simulink library "wt_blockset_beta"  (Simulink 5.0)
values from neighbouring files (symbols this model uses):
  a = -Le\Re    [matrix_coeff_trafo3limb_abc.m]
  a11 = K2*Rs/Ls    [matrix_coeff_scim_abc.m]    (also in matrix_coeff_spsm_dq.m = -Rs*Ksgm_frd/Ksgm_d; matrix_coeff_trafo_abc.m = K2*Rhv/Lhv; matrix_coeff_wrim_abc.m)
  a12 = K3*Rs/Ls    [matrix_coeff_scim_abc.m]    (also in matrix_coeff_spsm_dq.m = Lssq*Ksgm_frd/Ksgm_d; matrix_coeff_trafo_abc.m = K3*Rhv/Lhv; matrix_coeff_wrim_abc.m)
  a13 = 3*Msr*sqrt(3)*K4/4    [matrix_coeff_scim_abc.m]    (also in matrix_coeff_spsm_dq.m = Rf*Lsgm_rd*Lmd/Ksgm_d; matrix_coeff_trafo_abc.m = K4*Rhv; matrix_coeff_wrim_abc.m)
  a14 = K4*Rr    [matrix_coeff_scim_abc.m]    (also in matrix_coeff_spsm_dq.m = Rrd*Lsgm_f*Lmd/Ksgm_d; matrix_coeff_trafo_abc.m = K2/Lhv; matrix_coeff_wrim_abc.m)
  a15 = Msr*(K2-K3)/Ls    [matrix_coeff_scim_abc.m]    (also in matrix_coeff_spsm_dq.m = Lmq*Ksgm_frd/Ksgm_d; matrix_coeff_trafo_abc.m = K3/Lhv; matrix_coeff_wrim_abc.m)
  a16 = K2/Ls    [matrix_coeff_scim_abc.m]    (also in matrix_coeff_spsm_dq.m = Ksgm_frd/Ksgm_d; matrix_coeff_trafo_abc.m = K4; matrix_coeff_wrim_abc.m)
  a17 = K3/Ls    [matrix_coeff_scim_abc.m]    (also in matrix_coeff_spsm_dq.m = -Lsgm_rd*Lmd/Ksgm_d; matrix_coeff_wrim_abc.m)
  a21 = -Lssd*Lsrq/Ksgm_q    [matrix_coeff_spsm_dq.m]
  a22 = -Rs*Lsrq/Ksgm_q    [matrix_coeff_spsm_dq.m]
  a23 = -Lsrq*Lmd/Ksgm_q    [matrix_coeff_spsm_dq.m]
  a24 = -Lsrq*Lmd/Ksgm_q    [matrix_coeff_spsm_dq.m]
  a25 = Rrq*Lmq/Ksgm_q    [matrix_coeff_spsm_dq.m]
  a26 = Lsrq/Ksgm_q    [matrix_coeff_spsm_dq.m]
  a31 = K4*Rs    [matrix_coeff_scim_abc.m]    (also in matrix_coeff_spsm_dq.m = +Rs*Lsgm_rd*Lmd/Ksgm_d; matrix_coeff_trafo_abc.m = K4*Rlv; matrix_coeff_wrim_abc.m)
  a32 = Msr*(K2-K3)/Lr    [matrix_coeff_scim_abc.m]    (also in matrix_coeff_spsm_dq.m = -Lssq*Lsgm_rd*Lmd/Ksgm_d; matrix_coeff_trafo_abc.m = K2*Rlv/Llv; matrix_coeff_wrim_abc.m)
  a33 = K2*Rr/Lr    [matrix_coeff_scim_abc.m]    (also in matrix_coeff_spsm_dq.m = -Rf*Ksgm_srd/Ksgm_d; matrix_coeff_trafo_abc.m = K3*Rlv/Llv; matrix_coeff_wrim_abc.m)
  a34 = K3*Rr/Lr    [matrix_coeff_scim_abc.m]    (also in matrix_coeff_spsm_dq.m = Rrd*Lsgm_s*Lmd/Ksgm_d; matrix_coeff_trafo_abc.m = K4; matrix_coeff_wrim_abc.m)
  a35 = 3*Msr*sqrt(3)*K4/4    [matrix_coeff_scim_abc.m]    (also in matrix_coeff_spsm_dq.m = -Lsgm_rd*Lmd*Lmq/Ksgm_d; matrix_coeff_trafo_abc.m = K2/Llv; matrix_coeff_wrim_abc.m)
  a36 = K4    [matrix_coeff_scim_abc.m]    (also in matrix_coeff_spsm_dq.m = -Lsgm_rd*Lmd/Ksgm_d; matrix_coeff_trafo_abc.m = K3/Llv; matrix_coeff_wrim_abc.m)
  a37 = Ksgm_srd/Ksgm_d    [matrix_coeff_spsm_dq.m]    (also in matrix_coeff_wrim_abc.m = K2/Lr)
  a41 = Rs*Lsgm_f*Lmd/Ksgm_d    [matrix_coeff_spsm_dq.m]
  a42 = -Lsgm_f*Lssq*Lmd/Ksgm_d    [matrix_coeff_spsm_dq.m]
  a43 = Rf*Lsgm_s*Lmd/Ksgm_d    [matrix_coeff_spsm_dq.m]
  a44 = -Rrd*Ksgm_sf/Ksgm_d    [matrix_coeff_spsm_dq.m]
  a45 = -Lsgm_f*Lmd*Lmq/Ksgm_d    [matrix_coeff_spsm_dq.m]
  a46 = -Lsgm_f*Lmd/Ksgm_d    [matrix_coeff_spsm_dq.m]
  a47 = -Lsgm_s*Lmd/Ksgm_d    [matrix_coeff_spsm_dq.m]
  a51 = Lssd*Lmq/Ksgm_q    [matrix_coeff_spsm_dq.m]
  a52 = Rs*Lmq/Ksgm_q    [matrix_coeff_spsm_dq.m]
  a53 = Lmd*Lmq/Ksgm_q    [matrix_coeff_spsm_dq.m]
  a54 = Lmd*Lmq/Ksgm_q    [matrix_coeff_spsm_dq.m]
  a55 = -Rrq*Lssq/Ksgm_q    [matrix_coeff_spsm_dq.m]
  a56 = -Lmq/Ksgm_q    [matrix_coeff_spsm_dq.m]
  alpha_T = Ubase_hv/Ubase_lv    [matrix_coeff_trafo3limb_abc.m]
  b = inv(Le)    [matrix_coeff_trafo3limb_abc.m]
  Ctorque = cq(2:5:102,2:5:182)    [cq_table.m]
  Lmd = mag_ind(1)    [matrix_coeff_spsm_dq.m]
  Lmq = mag_ind(2)    [matrix_coeff_spsm_dq.m]
  Lss = Lsgms+Lm    [init_dbe_dq_scim.m]
  omg_base = 2*pi*rated_fp(1)    [init_dbe_dq_scim.m]    (also in init_dbe_rms_scim.m)
  p = rated_fp(2)    [init_dbe_dq_scim.m]    (also in init_dbe_rms_scim.m)
  Rs = stator(1)    [init_dbe_dq_scim.m]    (also in init_dbe_rms_scim.m; matrix_coeff_scim_abc.m; matrix_coeff_spsm_dq.m = stator_winding(1); matrix_coeff_wrim_abc.m)
  Xs = omg_base*Lss    [init_dbe_dq_scim.m]    (also in init_dbe_rms_scim.m = Xsgm_s+Xm)
undefined symbols (not defined in the file or in its folder): get, j, Kmode, ModeOp, Type, u0
libraries: simulink_extras x12, simulink x4, dspinverses x1, dspmtrx3 x1, dspsigattribs x1, dspspect3 x1
(part 3 of 4)

== system wt_blockset_beta/Mechanical Components/Wind Model SB-2/3rd_Harmonic_Filter2 ==
  avg_wind : Inport
  in_1 : Inport  Port=2
  3rd harmonic Filter : Subsystem
  Unit Delay : UnitDelay  SampleTime=T_sample
  out_1 : Outport
  wires:
  3rd harmonic Filter/1(Out) -> out_1/1
  avg_wind/1 -> 3rd harmonic Filter/1(avg_wind)
  in_1/1 -> Unit Delay/1
  Unit Delay/1 -> 3rd harmonic Filter/2(In)

== system wt_blockset_beta/Mechanical Components/Wind Model SB-2/Kaimal_Filter_1 ==
  in_1 : Inport
  avg_wind : Inport  Port=2
  Fcn : Fcn  Expr=turb_int*sqrt(L*u(1))/100/sqrt(2)
  Kaimal Filter : Subsystem
  Product : Product  SaturateOnIntegerOverflow=on
  Unit Delay : UnitDelay  SampleTime=T_sample
  out_1 : Outport
  wires:
  Unit Delay/1 -> Kaimal Filter/2(In)
  in_1/1 -> Unit Delay/1
  avg_wind/1 -> Kaimal Filter/1(avg_wind), Fcn/1
  Fcn/1 -> Product/1
  Kaimal Filter/1(Out) -> Product/2
  Product/1 -> out_1/1

== system wt_blockset_beta/Mechanical Components/Wind Model SB-2/Kaimal_Filter_2 ==
  avg_wind : Inport
  in_1 : Inport  Port=2
  Fcn : Fcn  Expr=turb_int*sqrt(L*u(1))/100/sqrt(2)
  Kaimal Filter : Subsystem
  Product : Product  SaturateOnIntegerOverflow=on
  Unit Delay : UnitDelay  SampleTime=T_sample
  out_1 : Outport
  wires:
  Product/1 -> out_1/1
  Kaimal Filter/1(Out) -> Product/2
  Fcn/1 -> Product/1
  avg_wind/1 -> Fcn/1, Kaimal Filter/1(avg_wind)
  in_1/1 -> Unit Delay/1
  Unit Delay/1 -> Kaimal Filter/2(In)

== system wt_blockset_beta/Mechanical Components/Wind Model SB-2/Kaimal_Filter_3 ==
  avg_wind : Inport
  in_1 : Inport  Port=2
  Fcn : Fcn  Expr=turb_int*sqrt(L*u(1))/100/sqrt(2)
  Kaimal Filter : Subsystem
  Product : Product  SaturateOnIntegerOverflow=on
  Unit Delay : UnitDelay  SampleTime=T_sample
  out_1 : Outport
  wires:
  Unit Delay/1 -> Kaimal Filter/2(In)
  in_1/1 -> Unit Delay/1
  avg_wind/1 -> Kaimal Filter/1(avg_wind), Fcn/1
  Fcn/1 -> Product/1
  Kaimal Filter/1(Out) -> Product/2
  Product/1 -> out_1/1

== system wt_blockset_beta/Mechanical Components/Wind Model SB-2/White Noise_1 ==
  Gain : Gain  Gain=[sqrt(Cov)]/[sqrt(Ts)]  SaturateOnIntegerOverflow=on
  White Noise : RandomNumber  Seed=seed  SampleTime=Ts
  Zero-Order Hold : ZeroOrderHold  SampleTime=Ts
  Out_1 : Outport
  wires:
  Zero-Order Hold/1 -> Gain/1
  Gain/1 -> Out_1/1
  White Noise/1 -> Zero-Order Hold/1

== system wt_blockset_beta/Mechanical Components/Wind Model SB-2/White Noise_2 ==
  Gain : Gain  Gain=[sqrt(Cov)]/[sqrt(Ts)]  SaturateOnIntegerOverflow=on
  White Noise : RandomNumber  Seed=seed  SampleTime=Ts
  Zero-Order Hold : ZeroOrderHold  SampleTime=Ts
  Out_1 : Outport
  wires:
  Zero-Order Hold/1 -> Gain/1
  Gain/1 -> Out_1/1
  White Noise/1 -> Zero-Order Hold/1

== system wt_blockset_beta/Mechanical Components/Wind Model SB-2/White Noise_3 ==
  Gain : Gain  Gain=[sqrt(Cov)]/[sqrt(Ts)]  SaturateOnIntegerOverflow=on
  White Noise : RandomNumber  Seed=seed  SampleTime=Ts
  Zero-Order Hold : ZeroOrderHold  SampleTime=Ts
  Out_1 : Outport
  wires:
  Zero-Order Hold/1 -> Gain/1
  Gain/1 -> Out_1/1
  White Noise/1 -> Zero-Order Hold/1

== system wt_blockset_beta/Mechanical Components/Wind Model SB-2/ZERO_Harmonic_Filter ==
  in_1 : Inport
  avg_wind : Inport  Port=2
  Unit Delay : UnitDelay  SampleTime=T_sample
  ZERO harmonic Filter : Subsystem
  out_1 : Outport
  wires:
  ZERO harmonic Filter/1(Out) -> out_1/1
  avg_wind/1 -> ZERO harmonic Filter/1(avg_wind)
  in_1/1 -> Unit Delay/1
  Unit Delay/1 -> ZERO harmonic Filter/2(In)

== system wt_blockset_beta/Power Converters/3-phase Diode Bridge Rectifier/Diode  State Calculator ==
  note: K = [d1 - d4
      |        d3 - d6
      |         d5 - d2]
  RST : Inport
  Branch A+ : Subsystem
  Branch A- : Subsystem
  Branch B+ : Subsystem
  Branch B- : Subsystem
  Branch C+ : Subsystem
  Branch C- : Subsystem
  Mux : Mux  Inputs=3
  Sum : Sum  Inputs=+-  SaturateOnIntegerOverflow=on  InputSameDT=on
  Sum1 : Sum  Inputs=+-  SaturateOnIntegerOverflow=on  InputSameDT=on
  Sum2 : Sum  Inputs=+-  SaturateOnIntegerOverflow=on  InputSameDT=on
  K : Outport  InitialOutput=0
  wires:
  RST/1 -> Branch A+/1(RST), Branch B+/1(RST), Branch B-/1(RST), Branch C+/1(RST), Branch C-/1(RST), Branch A-/1(RST)
  Branch A+/1(A) -> Sum/1
  Branch A-/1(A) -> Sum/2
  Branch B+/1(B) -> Sum1/1
  Branch B-/1(B) -> Sum1/2
  Branch C+/1(C) -> Sum2/1
  Branch C-/1(C) -> Sum2/2
  Sum/1 -> Mux/1
  Sum1/1 -> Mux/2
  Sum2/1 -> Mux/3
  Mux/1 -> K/1

== system wt_blockset_beta/Power Converters/Average SVM Strategy/1st quadrant ==
  note: 1st quadrant
  vd : Inport
  vq : Inport  Port=2
  Action Port : ActionPort  InitializeStates=reset
  Gain : Gain  Gain=sqrt(3)  SaturateOnIntegerOverflow=on
  If : If  NumInputs=2  IfExpression=u2 < u1
  Sector 0 : Subsystem  TreatAsAtomicUnit=on
  Sector 1 : Subsystem  TreatAsAtomicUnit=on
  Sum : Sum  Inputs=+|+  SaturateOnIntegerOverflow=on
  duty_ABC : Outport  OutputWhenDisabled=reset  InitialOutput=[0 0 0]
  wires:
  vd/1 -> Gain/1, [vd]
  vq/1 -> If/2, [vq]
  Gain/1 -> If/1
  If/1 -> Sector 0/Action
  [vd] -> Sector 0/1(vd)
  [vq] -> Sector 0/2(vq)
  If/2 -> Sector 1/Action
  [vd] -> Sector 1/1(vd)
  [vq] -> Sector 1/2(vq)
  Sector 1/1(duty_ABC) -> Sum/2
  Sector 0/1(duty_ABC) -> Sum/1
  Sum/1 -> duty_ABC/1

== system wt_blockset_beta/Power Converters/Average SVM Strategy/2nd quadrant ==
  note: 2nd quadrant
  vd : Inport
  vq : Inport  Port=2
  Action Port : ActionPort  InitializeStates=reset
  Abs : Abs  SaturateOnIntegerOverflow=on
  Gain : Gain  Gain=sqrt(3)  SaturateOnIntegerOverflow=on
  If : If  NumInputs=2  IfExpression=u2 < u1
  Sector 1 : Subsystem  TreatAsAtomicUnit=on
  Sector 2 : Subsystem  TreatAsAtomicUnit=on
  Sum : Sum  Inputs=+|+  SaturateOnIntegerOverflow=on
  duty_ABC : Outport  OutputWhenDisabled=reset  InitialOutput=[0 0 0]
  wires:
  Sum/1 -> duty_ABC/1
  Sector 2/1(duty_ABC) -> Sum/1
  Sector 1/1(duty_ABC) -> Sum/2
  [vq] -> Sector 1/2(vq)
  [vd] -> Sector 1/1(vd)
  If/2 -> Sector 1/Action
  [vq] -> Sector 2/2(vq)
  [vd] -> Sector 2/1(vd)
  If/1 -> Sector 2/Action
  vq/1 -> [vq], If/2
  vd/1 -> [vd], Abs/1
  Gain/1 -> If/1
  Abs/1 -> Gain/1

== system wt_blockset_beta/Power Converters/Average SVM Strategy/3rd quadrant ==
  note: 3rd quadrant
  vd : Inport
  vq : Inport  Port=2
  Action Port : ActionPort  InitializeStates=reset
  Abs : Abs  SaturateOnIntegerOverflow=on
  Abs1 : Abs  SaturateOnIntegerOverflow=on
  Gain : Gain  Gain=sqrt(3)  SaturateOnIntegerOverflow=on
  If : If  NumInputs=2  IfExpression=u2 <= u1
  Sector 3 : Subsystem  TreatAsAtomicUnit=on
  Sector 4 : Subsystem  TreatAsAtomicUnit=on
  Sum : Sum  Inputs=+|+  SaturateOnIntegerOverflow=on
  duty_ABC : Outport  OutputWhenDisabled=reset  InitialOutput=[0 0 0]
  wires:
  Sum/1 -> duty_ABC/1
  Sector 3/1(duty_ABC) -> Sum/1
  Sector 4/1(duty_ABC) -> Sum/2
  [vq] -> Sector 4/2(vq)
  [vd] -> Sector 4/1(vd)
  If/2 -> Sector 4/Action
  [vq] -> Sector 3/2(vq)
  [vd] -> Sector 3/1(vd)
  If/1 -> Sector 3/Action
  vq/1 -> [vq], Abs1/1
  vd/1 -> [vd], Abs/1
  Gain/1 -> If/1
  Abs/1 -> Gain/1
  Abs1/1 -> If/2

== system wt_blockset_beta/Power Converters/Average SVM Strategy/4th quadrant ==
  note: 4th quadrant
  vd : Inport
  vq : Inport  Port=2
  Action Port : ActionPort  InitializeStates=reset
  Abs1 : Abs  SaturateOnIntegerOverflow=on
  Gain : Gain  Gain=sqrt(3)  SaturateOnIntegerOverflow=on
  If : If  NumInputs=2  IfExpression=u2 <= u1
  Sector 4 : Subsystem  TreatAsAtomicUnit=on
  Sector 5 : Subsystem  TreatAsAtomicUnit=on
  Sum : Sum  Inputs=+|+  SaturateOnIntegerOverflow=on
  duty_ABC : Outport  OutputWhenDisabled=reset  InitialOutput=[0 0 0]
  wires:
  Abs1/1 -> If/2
  vd/1 -> [vd], Gain/1
  vq/1 -> Abs1/1, [vq]
  If/1 -> Sector 5/Action
  [vd] -> Sector 5/1(vd)
  [vq] -> Sector 5/2(vq)
  If/2 -> Sector 4/Action
  [vd] -> Sector 4/1(vd)
  [vq] -> Sector 4/2(vq)
  Sector 4/1(duty_ABC) -> Sum/2
  Sector 5/1(duty_ABC) -> Sum/1
  Sum/1 -> duty_ABC/1
  Gain/1 -> If/1

== system wt_blockset_beta/Power Converters/Average SVM Strategy/Avoid saturation  ==
  Mux : Mux  Inputs=7
  Sign_vdref : Signum
  Sign_vqref : Signum
  vd : Fcn  Expr=(abs(u[1])>u[6])*((3*u(2)*u[6])/(2*u[5]))+(abs(u[1])<=u[6])*(3*u[1]/2/u[5])
  vq : Fcn  Expr=(abs(u[3])>u[7])*((3*u(4)*u[7])/(2*u[5]))+(abs(u[3])<=u[7])*(3*u[3]/2/u[5])
  tag scope: vd=global, vq=global
  wires:
  [vdref] -> Mux/1, Sign_vdref/1
  Mux/1 -> vd/1, vq/1
  vd/1 -> [vd]
  vq/1 -> [vq]
  Sign_vdref/1 -> Mux/2
  [vqref] -> Mux/3, Sign_vqref/1
  Sign_vqref/1 -> Mux/4
  [vdc] -> Mux/5
  [dlim] -> Mux/6
  [qlim] -> Mux/7

== system wt_blockset_beta/Power Converters/Average SVM Strategy/Weight ==
  Abs : Abs  SaturateOnIntegerOverflow=on
  "Abs " : Abs  SaturateOnIntegerOverflow=on
  Mux : Mux  Inputs=3
  Product : Product  SaturateOnIntegerOverflow=on
  Product1 : Product  SaturateOnIntegerOverflow=on
  weight : Fcn  Expr=u(2)/(sqrt(3)*sqrt(u(1)^2+u(3)^2))
  tag scope: dlim=global, qlim=global
  wires:
  [vdref] -> Mux/1, Product/1
  Mux/1 -> weight/1
  [vdc] -> Mux/2
  [vqref] -> Mux/3, Product1/2
  weight/1 -> Product/2, Product1/1
  Product/1 -> Abs/1
  Product1/1 -> "Abs "/1
  Abs/1 -> [dlim]
  "Abs "/1 -> [qlim]

== system wt_blockset_beta/Power Converters/Average SVM Strategy/capcom duty cycle ==
  duty_ABC : Inport
  Constant : Constant  Value=0.5
  Sum : Sum  Inputs=|+-  SaturateOnIntegerOverflow=on
  pwm_abc : Outport
  wires:
  Constant/1 -> Sum/2
  Sum/1 -> pwm_abc/1
  duty_ABC/1 -> Sum/1

== system wt_blockset_beta/Power Converters/Switching PWM Strategy/capcom ==
  duty_abc : Inport
  Reshape : simulink/Math Operations/Reshape  OutputDimensionality=1-D array  OutputDimensions=[1,1]
  Sum : Sum  Inputs=-+  SaturateOnIntegerOverflow=on  InputSameDT=on
  Vtri1 : Subsystem  mask{fsw=carrier}
      mask prompts: fsw "switching frequency"
      mask init:
      | fsw2=fsw*2;
      | x=[0 1/4 3/4 1];
      | y=[0 -1     1    0];
      mask Display: plot([x  x+1 ],[y y])
  pulses : Subsystem
      mask init:
      | x=[-5 0 0 5];
      | y=[ 0 0 1 1];
      mask Display: plot(x,y)
  S_ABC : Outport
  wires:
  Reshape/1 -> S_ABC/1  "q"
  Sum/1 -> pulses/1(In1)
  duty_abc/1 -> Sum/2  "Vcontrol"
  Vtri1/1(Vtri) -> Sum/1  "Vtri"
  pulses/1(Out1) -> Reshape/1  "q"

== system wt_blockset_beta/Power Converters/Switching PWM Strategy/dead_time_A ==
  pwm_A : Inport
  Data Type Conversion : DataTypeConversion  DataType=double  SaturateOnIntegerOverflow=on
  Data Type Conversion1 : DataTypeConversion  DataType=boolean  SaturateOnIntegerOverflow=on
  Data Type Conversion2 : DataTypeConversion  DataType=boolean  SaturateOnIntegerOverflow=on
  Logical Operator : Logic
  Transport Delay : TransportDelay  DelayTime=dead_time  BufferSize=8192
  S_A : Outport
  wires:
  Logical Operator/1 -> Data Type Conversion/1
  pwm_A/1 -> Transport Delay/1, Data Type Conversion1/1
  Transport Delay/1 -> Data Type Conversion2/1
  Data Type Conversion/1 -> S_A/1
  Data Type Conversion1/1 -> Logical Operator/1
  Data Type Conversion2/1 -> Logical Operator/2

== system wt_blockset_beta/Power Converters/Switching PWM Strategy/pulse dropping ==
  duty_ABC : Inport
  A : Fcn  Expr=(mpw*(u(1)<=mpw)+u(1)*(u(1)>mpw))*(dp==0)+u(1)*(dp==1)
  B : Fcn  Expr=(mpw*(u(2)<=mpw)+u(2)*(u(2)>mpw))*(dp==0)+u(2)*(dp==1)
  C : Fcn  Expr=(mpw*(u(3)<=mpw)+u(3)*(u(3)>mpw))*(dp==0)+u(3)*(dp==1)
  Mux2 : Mux  Inputs=3
  duty_abc : Outport
  wires:
  A/1 -> Mux2/1
  Mux2/1 -> duty_abc/1
  duty_ABC/1 -> A/1, B/1, C/1
  B/1 -> Mux2/2
  C/1 -> Mux2/3

== system wt_blockset_beta/Power Converters/Switching SVM Strategy/1st quadrant ==
  note: 1st quadrant
  vd : Inport
  vq : Inport  Port=2
  Action Port : ActionPort  InitializeStates=reset
  Gain : Gain  Gain=sqrt(3)  SaturateOnIntegerOverflow=on
  If : If  NumInputs=2  IfExpression=u2 < u1
  Sector 0 : Subsystem  TreatAsAtomicUnit=on
  Sector 1 : Subsystem  TreatAsAtomicUnit=on
  Sum : Sum  Inputs=+|+  SaturateOnIntegerOverflow=on
  duty_ABC : Outport  OutputWhenDisabled=reset  InitialOutput=[0 0 0]
  wires:
  vd/1 -> Gain/1, [vd]
  vq/1 -> If/2, [vq]
  Gain/1 -> If/1
  If/1 -> Sector 0/Action
  [vd] -> Sector 0/1(vd)
  [vq] -> Sector 0/2(vq)
  If/2 -> Sector 1/Action
  [vd] -> Sector 1/1(vd)
  [vq] -> Sector 1/2(vq)
  Sector 1/1(duty_ABC) -> Sum/2
  Sector 0/1(duty_ABC) -> Sum/1
  Sum/1 -> duty_ABC/1

== system wt_blockset_beta/Power Converters/Switching SVM Strategy/2nd quadrant ==
  note: 2nd quadrant
  vd : Inport
  vq : Inport  Port=2
  Action Port : ActionPort  InitializeStates=reset
  Abs : Abs  SaturateOnIntegerOverflow=on
  Gain : Gain  Gain=sqrt(3)  SaturateOnIntegerOverflow=on
  If : If  NumInputs=2  IfExpression=u2 < u1
  Sector 1 : Subsystem  TreatAsAtomicUnit=on
  Sector 2 : Subsystem  TreatAsAtomicUnit=on
  Sum : Sum  Inputs=+|+  SaturateOnIntegerOverflow=on
  duty_ABC : Outport  OutputWhenDisabled=reset  InitialOutput=[0 0 0]
  wires:
  Sum/1 -> duty_ABC/1
  Sector 2/1(duty_ABC) -> Sum/1
  Sector 1/1(duty_ABC) -> Sum/2
  [vq] -> Sector 1/2(vq)
  [vd] -> Sector 1/1(vd)
  If/2 -> Sector 1/Action
  [vq] -> Sector 2/2(vq)
  [vd] -> Sector 2/1(vd)
  If/1 -> Sector 2/Action
  vq/1 -> [vq], If/2
  vd/1 -> [vd], Abs/1
  Gain/1 -> If/1
  Abs/1 -> Gain/1

== system wt_blockset_beta/Power Converters/Switching SVM Strategy/3rd quadrant ==
  note: 3rd quadrant
  vd : Inport
  vq : Inport  Port=2
  Action Port : ActionPort  InitializeStates=reset
  Abs : Abs  SaturateOnIntegerOverflow=on
  Abs1 : Abs  SaturateOnIntegerOverflow=on
  Gain : Gain  Gain=sqrt(3)  SaturateOnIntegerOverflow=on
  If : If  NumInputs=2  IfExpression=u2 <= u1
  Sector 3 : Subsystem  TreatAsAtomicUnit=on
  Sector 4 : Subsystem  TreatAsAtomicUnit=on
  Sum : Sum  Inputs=+|+  SaturateOnIntegerOverflow=on
  duty_ABC : Outport  OutputWhenDisabled=reset  InitialOutput=[0 0 0]
  wires:
  Sum/1 -> duty_ABC/1
  Sector 3/1(duty_ABC) -> Sum/1
  Sector 4/1(duty_ABC) -> Sum/2
  [vq] -> Sector 4/2(vq)
  [vd] -> Sector 4/1(vd)
  If/2 -> Sector 4/Action
  [vq] -> Sector 3/2(vq)
  [vd] -> Sector 3/1(vd)
  If/1 -> Sector 3/Action
  vq/1 -> [vq], Abs1/1
  vd/1 -> [vd], Abs/1
  Gain/1 -> If/1
  Abs/1 -> Gain/1
  Abs1/1 -> If/2

== system wt_blockset_beta/Power Converters/Switching SVM Strategy/4th quadrant ==
  note: 4th quadrant
  vd : Inport
  vq : Inport  Port=2
  Action Port : ActionPort  InitializeStates=reset
  Abs1 : Abs  SaturateOnIntegerOverflow=on
  Gain : Gain  Gain=sqrt(3)  SaturateOnIntegerOverflow=on
  If : If  NumInputs=2  IfExpression=u2 <= u1
  Sector 4 : Subsystem  TreatAsAtomicUnit=on
  Sector 5 : Subsystem  TreatAsAtomicUnit=on
  Sum : Sum  Inputs=+|+  SaturateOnIntegerOverflow=on
  duty_ABC : Outport  OutputWhenDisabled=reset  InitialOutput=[0 0 0]
  wires:
  Abs1/1 -> If/2
  vd/1 -> [vd], Gain/1
  vq/1 -> Abs1/1, [vq]
  If/1 -> Sector 5/Action
  [vd] -> Sector 5/1(vd)
  [vq] -> Sector 5/2(vq)
  If/2 -> Sector 4/Action
  [vd] -> Sector 4/1(vd)
  [vq] -> Sector 4/2(vq)
  Sector 4/1(duty_ABC) -> Sum/2
  Sector 5/1(duty_ABC) -> Sum/1
  Sum/1 -> duty_ABC/1
  Gain/1 -> If/1

== system wt_blockset_beta/Power Converters/Switching SVM Strategy/Avoid saturation  ==
  Mux : Mux  Inputs=7
  Sign_vdref : Signum
  Sign_vqref : Signum
  vd : Fcn  Expr=(abs(u[1])>u[6])*((3*u(2)*u[6])/(2*u[5]))+(abs(u[1])<=u[6])*(3*u[1]/2/u[5])
  vq : Fcn  Expr=(abs(u[3])>u[7])*((3*u(4)*u[7])/(2*u[5]))+(abs(u[3])<=u[7])*(3*u[3]/2/u[5])
  tag scope: vd=global, vq=global
  wires:
  [vdref] -> Mux/1, Sign_vdref/1
  Mux/1 -> vd/1, vq/1
  vd/1 -> [vd]
  vq/1 -> [vq]
  Sign_vdref/1 -> Mux/2
  [vqref] -> Mux/3, Sign_vqref/1
  Sign_vqref/1 -> Mux/4
  [vdc] -> Mux/5
  [dlim] -> Mux/6
  [qlim] -> Mux/7

== system wt_blockset_beta/Power Converters/Switching SVM Strategy/Weight ==
  Abs : Abs  SaturateOnIntegerOverflow=on
  "Abs " : Abs  SaturateOnIntegerOverflow=on
  Mux : Mux  Inputs=3
  Product : Product  SaturateOnIntegerOverflow=on
  Product1 : Product  SaturateOnIntegerOverflow=on
  weight : Fcn  Expr=u(2)/(sqrt(3)*sqrt(u(1)^2+u(3)^2))
  tag scope: dlim=global, qlim=global
  wires:
  [vdref] -> Mux/1, Product/1
  Mux/1 -> weight/1
  [vdc] -> Mux/2
  [vqref] -> Mux/3, Product1/2
  weight/1 -> Product/2, Product1/1
  Product/1 -> Abs/1
  Product1/1 -> "Abs "/1
  Abs/1 -> [dlim]
  "Abs "/1 -> [qlim]

== system wt_blockset_beta/Power Converters/Switching SVM Strategy/capcom duty cycle -> 0..1 ==
  duty_ABC : Inport
  Clock : Clock
  Math Function : Math  Operator=rem
  Mux : Mux  Inputs=[3 1]
  Mux2 : Mux  Inputs=3
  Switch_A : Fcn  Expr=(u[4]>=0.5*Tsw*(1-u[1]))*(u[4]<=0.5*Tsw*(1+u[1]))
  Switch_B : Fcn  Expr=(u(4)>=0.5*Tsw*(1-u(2)))*(u(4)<=0.5*Tsw*(1+u(2)))
  Switch_C : Fcn  Expr=(u(4)>=0.5*Tsw*(1-u(3)))*(u(4)<=0.5*Tsw*(1+u(3)))
  Tsw : Constant  Value=Tsw
  pwm_abc : Outport
  wires:
  Mux/1 -> Switch_C/1, Switch_A/1, Switch_B/1
  Math Function/1 -> Mux/2
  Clock/1 -> Math Function/1
  duty_ABC/1 -> Mux/1
  Tsw/1 -> Math Function/2
  Switch_A/1 -> Mux2/1
  Switch_B/1 -> Mux2/2
  Switch_C/1 -> Mux2/3
  Mux2/1 -> pwm_abc/1

== system wt_blockset_beta/Power Converters/Switching SVM Strategy/dead_time_ABC ==
  pwm_ABC : Inport
  Data Type Conversion : DataTypeConversion  DataType=double  SaturateOnIntegerOverflow=on
  Data Type Conversion1 : DataTypeConversion  DataType=boolean  SaturateOnIntegerOverflow=on
  Data Type Conversion2 : DataTypeConversion  DataType=boolean  SaturateOnIntegerOverflow=on
  Logical Operator : Logic
  Transport Delay : TransportDelay  DelayTime=dead_time  BufferSize=8192
  S_ABC : Outport
  wires:
  Logical Operator/1 -> Data Type Conversion/1
  pwm_ABC/1 -> Transport Delay/1, Data Type Conversion1/1
  Transport Delay/1 -> Data Type Conversion2/1
  Data Type Conversion/1 -> S_ABC/1
  Data Type Conversion1/1 -> Logical Operator/1
  Data Type Conversion2/1 -> Logical Operator/2

== system wt_blockset_beta/Power Converters/Switching SVM Strategy/pulse dropping ==
  duty_ABC : Inport
  A : Fcn  Expr=(mpw*(u(1)<=mpw)+u(1)*(u(1)>mpw))*(dp==0)+u(1)*(dp==1)
  B : Fcn  Expr=(mpw*(u(2)<=mpw)+u(2)*(u(2)>mpw))*(dp==0)+u(2)*(dp==1)
  C : Fcn  Expr=(mpw*(u(3)<=mpw)+u(3)*(u(3)>mpw))*(dp==0)+u(3)*(dp==1)
  Mux2 : Mux  Inputs=3
  duty_abc : Outport
  wires:
  A/1 -> Mux2/1
  Mux2/1 -> duty_abc/1
  duty_ABC/1 -> A/1, B/1, C/1
  B/1 -> Mux2/2
  C/1 -> Mux2/3

== system wt_blockset_beta/Common Models/Circuit breaker/Circuit breaker1/delay tc ==
  note: AND  used to suppress
      | spurious operation when
      | input goes from high to low
  in_1 : Inport
  Logical Operator : Logic  Operator=XOR
  Logical Operator1 : Logic
  Transport Delay1 : TransportDelay  DelayTime=tc  BufferSize=20000
  out_1 : Outport
  wires:
  Transport Delay1/1 -> Logical Operator/2
  in_1/1 -> Logical Operator/1, Transport Delay1/1, Logical Operator1/1
  Logical Operator1/1 -> out_1/1
  Logical Operator/1 -> Logical Operator1/2

== system wt_blockset_beta/Common Models/Circuit breaker/Circuit breaker2/delay tc ==
  note: AND  used to suppress
      | spurious operation when
      | input goes from high to low
  in_1 : Inport
  Logical Operator : Logic  Operator=XOR
  Logical Operator1 : Logic
  Transport Delay1 : TransportDelay  DelayTime=tc  BufferSize=20000
  out_1 : Outport
  wires:
  Logical Operator/1 -> Logical Operator1/2
  Logical Operator1/1 -> out_1/1
  in_1/1 -> Logical Operator1/1, Transport Delay1/1, Logical Operator/1
  Transport Delay1/1 -> Logical Operator/2

== system wt_blockset_beta/Common Models/Circuit breaker/Circuit breaker3/delay tc ==
  note: AND  used to suppress
      | spurious operation when
      | input goes from high to low
  in_1 : Inport
  Logical Operator : Logic  Operator=XOR
  Logical Operator1 : Logic
  Transport Delay1 : TransportDelay  DelayTime=tc  BufferSize=20000
  out_1 : Outport
  wires:
  Transport Delay1/1 -> Logical Operator/2
  in_1/1 -> Logical Operator/1, Transport Delay1/1, Logical Operator1/1
  Logical Operator1/1 -> out_1/1
  Logical Operator/1 -> Logical Operator1/2

== system wt_blockset_beta/Electrical Machinery/Simulink Blocks  based Models/RMS Wound Rotor Induction Machine/Impedance Matrix ==
  omg : Inport
  Matrix Concatenation1 : simulink/Math Operations/Matrix Concatenation  numInports=2  catMethod=Horizontal
  Matrix Concatenation2 : simulink/Math Operations/Matrix Concatenation  numInports=2  catMethod=Horizontal
  Matrix Concatenation3 : simulink/Math Operations/Matrix Concatenation  numInports=2  catMethod=Vertical
  Product : Product  SaturateOnIntegerOverflow=on  InputSameDT=on
  Product1 : Product  SaturateOnIntegerOverflow=on  InputSameDT=on
  Real-Imag to Complex{,1..3} (4 alike) : RealImagToComplex
  Rs : Constant  Value=Rs
  Xm : Constant  Value=Xm
  Xm1 : Constant  Value=Xm
  Xs : Constant  Value=Xs
  d : Constant  Value=0
  d1 : Constant  Value=0
  rotor reactance : Fcn  Expr=Xsgm_r*(abs(u(1))<=sbd)+(Xsgm_r*((kx-1)*abs(u(1))+(1-kx*sbd))/(1-sbd))*(abs(u(1))>sbd)+Xm
  rotor resistance : Fcn  Expr=Rr*(abs(u(1))<=sbd)+(Rr*((kr-1)*abs(u(1))+(1-kr*sbd))/(1-sbd))*(abs(u(1))>sbd)
  slip : Fcn  Expr=1-u(1)/omg_synch
  Z : Outport
  wires:
  Matrix Concatenation3/1 -> Z/1
  Matrix Concatenation1/1 -> Matrix Concatenation3/1
  Matrix Concatenation2/1 -> Matrix Concatenation3/2
  Real-Imag to Complex2/1 -> Matrix Concatenation2/2
  Real-Imag to Complex3/1 -> Matrix Concatenation2/1
  Xm1/1 -> Product1/1
  Product1/1 -> Real-Imag to Complex3/2
  d1/1 -> Real-Imag to Complex3/1
  Product/1 -> Real-Imag to Complex2/2
  d/1 -> Real-Imag to Complex1/1
  Real-Imag to Complex1/1 -> Matrix Concatenation1/2
  Real-Imag to Complex/1 -> Matrix Concatenation1/1
  Xm/1 -> Real-Imag to Complex1/2
  Xs/1 -> Real-Imag to Complex/2
  Rs/1 -> Real-Imag to Complex/1
  rotor resistance/1 -> Real-Imag to Complex2/1  "Rr"
  omg/1 -> slip/1  "slip"
  slip/1 -> Product1/2, Product/2, rotor reactance/1, rotor resistance/1
  rotor reactance/1 -> Product/1  "Xr"

== system wt_blockset_beta/Electrical Machinery/Simulink Blocks  based Models/RMS  Squirrel Cage Induction Machine/Steady State Model ==
  Vs : Inport
  omg : Inport  Port=2
  Complex to Magnitude-Angle : ComplexToMagnitudeAngle
  Mux : Mux
  Mux1 : Mux  Inputs=2
  Product : Product  Inputs=*/  SaturateOnIntegerOverflow=on  InputSameDT=on
  Real-Imag to Complex : RealImagToComplex
  Selector : Selector  Elements=[1]  InputPortWidth=4
  electromagnetique torque : Fcn  Expr=3*p*Xm^2*u(1)^2*u(2)*u(3)/((Rs*u(3)+(Xm^2-Xs*u(4))*u(2))^2+(u(3)*Xs+u(2)*Rs*u(4))^2)/omg_base
  equivalent reactance : Fcn  Expr=(((u(3)/u(2))^2)*Xs-u(4)*(Xm^2-Xs*u(4)))/((u(3)/u(2))^2+u(4)^2)
  equivalent resistance : Fcn  Expr=(Rs*(u(3)/u(2))^2+Xm^2*u(3)/u(2)+Rs*u(4))/((u(3)/u(2))^2+u(4)^2)
  m<->g : Fcn  Expr=u(1)*(u(2) >=0)-(pi-u(1))*(u(2) < 0)
  rad->deg : Gain  Gain=180/pi  SaturateOnIntegerOverflow=on
  rotor reactance : Fcn  Expr=Xsgm_r*(abs(u(1))<=sbd)+(Xsgm_r*((kx-1)*abs(u(1))+(1-kx*sbd))/(1-sbd))*(abs(u(1))>sbd)+Xm
  rotor resistance : Fcn  Expr=Rr*(abs(u(1))<=sbd)+(Rr*((kr-1)*abs(u(1))+(1-kr*sbd))/(1-sbd))*(abs(u(1))>sbd)
  slip : Fcn  Expr=1-u(1)/omg_base
  Te : Outport
  Iph : Outport  Port=2
  phase_angle : Outport  Port=3
  wires:
  m<->g/1 -> rad->deg/1
  Mux1/1 -> m<->g/1
  Complex to Magnitude-Angle/2 -> Mux1/1
  Real-Imag to Complex/1 -> Complex to Magnitude-Angle/1
  Product/1 -> Iph/1
  Selector/1 -> Product/1
  Complex to Magnitude-Angle/1 -> Product/2
  rad->deg/1 -> phase_angle/1
  equivalent reactance/1 -> Real-Imag to Complex/2
  equivalent resistance/1 -> Real-Imag to Complex/1
  Mux/1 -> equivalent reactance/1, Selector/1, electromagnetique torque/1, equivalent resistance/1
  rotor reactance/1 -> Mux/4
  electromagnetique torque/1 -> Te/1
  rotor resistance/1 -> Mux/3
  slip/1 -> Mux1/2, rotor reactance/1, rotor resistance/1, Mux/2
  Vs/1 -> Mux/1
  omg/1 -> slip/1

== system wt_blockset_beta/Electrical Machinery/Simulink Blocks  based Models/Salient-Pole Synchronous Machine constant parameters/Mathematical model ==
  usdq : Inport
  uf : Inport  Port=2
  omgr : Inport  Port=3
  Demux : Demux  Outputs=2
  Integrator{1..5} (5 alike) : Integrator
  Mux : Mux  Inputs=9
  Mux1 : Mux  Inputs=3
  Telm : Fcn  Expr=1.5*p*((Lmd-Lmq)*u[1]*u[2]+Lmq*u[2]*(u[3]+u[4])-Lmq*u[5]*u[1])
  dif/dt : Fcn  Expr=a31*u[1]+a32*u[9]*u[2]+a33*u[3]+a34*u[4]+a35*u[9]*u[5]+a36*u[6]+a37*u[8]
  dird/dt : Fcn  Expr=a41*u[1]+a42*u[9]*u[2]+a43*u[3]+a44*u[4]+a45*u[9]*u[5]+a46*u[6]+a47*u[8]
  dirq/dt : Fcn  Expr=a51*u[9]*u[1]+a52*u[2]+a53*u[9]*u[3]+a54*u[9]*u[4]+a55*u[5]+a56*u[7]
  disd/dt : Fcn  Expr=a11*u[1]+a12*u[9]*u[2]+a13*u[3]+a14*u[4]+a15*u[9]*u[5]+a16*u[6]+a17*u[8]
  disq/dt : Fcn  Expr=a21*u[9]*u[1]+a22*u[2]+a23*u[9]*u[3]+a24*u[9]*u[4]+a25*u[5]+a26*u[7]
  dq / abc : Subsystem
  isd : Selector  Elements=[1]  InputPortWidth=9
  isq : Selector  Elements=[2]  InputPortWidth=9
  Te : Outport  InitialOutput=0
  is_UVW : Outport  Port=2  InitialOutput=0
  wires:
  Mux/1 -> disd/dt/1, disq/dt/1, dif/dt/1, dird/dt/1, dirq/dt/1, Telm/1, isd/1, isq/1
  omgr/1 -> Mux/9
  uf/1 -> Mux/8
  disd/dt/1 -> Integrator4/1
  disq/dt/1 -> Integrator1/1
  dif/dt/1 -> Integrator2/1
  dird/dt/1 -> Integrator3/1
  dirq/dt/1 -> Integrator5/1
  Integrator5/1 -> Mux/5
  Integrator3/1 -> Mux/4
  Integrator2/1 -> Mux/3
  Integrator1/1 -> Mux/2
  Integrator4/1 -> Mux/1
  Telm/1 -> Te/1
  Demux/2 -> Mux/7
  Demux/1 -> Mux/6
  usdq/1 -> Demux/1
  dq / abc/1(A) -> Mux1/1
  dq / abc/2(B) -> Mux1/2
  dq / abc/3(C) -> Mux1/3
  Mux1/1 -> is_UVW/1
  [theta] -> dq / abc/3(theta)
  isd/1 -> dq / abc/1(D)
  isq/1 -> dq / abc/2(Q)

== system wt_blockset_beta/Electrical Machinery/Simulink Blocks  based Models/Salient-Pole Synchronous Machine constant parameters/abc-dq ==
  ABC : Inport
  theta : Inport  Port=2
  Mux : Mux  Inputs=[3 1]
  Mux1 : Mux  Inputs=2
  d : Fcn  Expr=2*(u[1]*cos(u[4])+u[2]*cos(u[4]-2*pi/3)+u[3]*cos(u[4]+2*pi/3))/3
  q : Fcn  Expr=-2*(u[1]*sin(u[4])+u[2]*sin(u[4]-2*pi/3)+u[3]*sin(u[4]+2*pi/3))/3
  DQ : Outport  InitialOutput=0
  wires:
  Mux/1 -> d/1, q/1
  ABC/1 -> Mux/1
  Mux1/1 -> DQ/1
  d/1 -> Mux1/1
  q/1 -> Mux1/2
  theta/1 -> Mux/2

== system wt_blockset_beta/Electrical Machinery/Simulink Blocks  based Models/Squirrel Cage Induction Machine constant parameters/Derivatives ==
  vdqs : Inport
  omega : Inport  Port=2
  Mux : Mux  Inputs=[1 1 1 1 2 1]
  Selector : Selector  Elements=[7]  InputPortWidth=7
  Selector1 : Selector  Elements=[1 2]  InputPortWidth=7
  didr/dt : Fcn  Expr=((Rs*Lm*u(1))/(Lss*Lsr)-Lm*u(7)*u(2)/Lsr-Rr*u(3)/Lsr-(Lm^2*u(7)*u(4))/(Lss*Lsr)-(Lm*u(5))/(Lss*Lsr))/sigma
  dids/dt : Fcn  Expr=(-Rs*u(1)/Lss+u(7)*u(2)+(Lm*Rr*u(3))/(Lss*Lsr)+Lm*u(7)*u(4)/Lss+u(5)/Lss)/sigma
  diqr/dt : Fcn  Expr=(Lm*u(7)*u(1)/Lsr+(Rs*Lm*u(2))/(Lss*Lsr)+(Lm^2*u(7)*u(3))/(Lss*Lsr)-Rr*u(4)/Lsr-(Lm*u(6))/(Lss*Lsr))/sigma
  diqs/dt : Fcn  Expr=(-u(7)*u(1)-Rs*u(2)/Lss-Lm*u(7)*u(3)/Lss+(Rr*Lm*u(4))/(Lss*Lsr)+u(6)/Lss)/sigma
  electromagnetique torque : Fcn  Expr=1.5*Lm*p*(u(2)*u(3)-u(1)*u(4))
  int_1 : Integrator  InitialCondition=x0(1)
  int_2 : Integrator  InitialCondition=x0(2)
  int_3 : Integrator  InitialCondition=x0(3)
  int_4 : Integrator  InitialCondition=x0(4)
  int_5 : Integrator  InitialCondition=x0(5)
  idqs : Outport
  Te : Outport  Port=2
  tag scope: theta=global
  wires:
  Selector1/1 -> idqs/1
  diqs/dt/1 -> int_2/1
  Selector/1 -> int_5/1
  int_5/1 -> [theta]  "theta"
  electromagnetique torque/1 -> Te/1
  diqr/dt/1 -> int_4/1
  didr/dt/1 -> int_3/1
  dids/dt/1 -> int_1/1
  Mux/1 -> Selector1/1, Selector/1, electromagnetique torque/1, diqr/dt/1, didr/dt/1, diqs/dt/1, dids/dt/1
  omega/1 -> Mux/6  "omega_rot"
  vdqs/1 -> Mux/5  "vdqs"
  int_4/1 -> Mux/4  "iqr"
  int_3/1 -> Mux/3  "idr"
  int_2/1 -> Mux/2  "iqs"
  int_1/1 -> Mux/1  "ids"

== system wt_blockset_beta/Electrical Machinery/Simulink Blocks  based Models/Squirrel Cage Induction Machine constant parameters/abc-dq ==
  ABC : Inport
  theta : Inport  Port=2
  Mux : Mux  Inputs=[3 1]
  Mux1 : Mux  Inputs=2
  d : Fcn  Expr=2*(u[1]*cos(u[4])+u[2]*cos(u[4]-2*pi/3)+u[3]*cos(u[4]+2*pi/3))/3
  q : Fcn  Expr=-2*(u[1]*sin(u[4])+u[2]*sin(u[4]-2*pi/3)+u[3]*sin(u[4]+2*pi/3))/3
  DQ : Outport  InitialOutput=0
  wires:
  q/1 -> Mux1/2  "vqs"
  theta/1 -> Mux/2
  Mux1/1 -> DQ/1
  d/1 -> Mux1/1  "vds"
  ABC/1 -> Mux/1
  Mux/1 -> q/1, d/1

== system wt_blockset_beta/Electrical Machinery/Simulink Blocks  based Models/Squirrel Cage Induction Machine constant parameters/dq / abc ==
  DQ : Inport
  theta : Inport  Port=2
  Mux : Mux  Inputs=[2 1]
  Mux1 : Mux  Inputs=3
  va : Fcn  Expr=u[1]*cos(u[3])-u[2]*sin(u[3])
  vb : Fcn  Expr=u[1]*cos(u[3]-2*pi/3)-u[2]*sin(u[3]-2*pi/3)
  vc : Fcn  Expr=u[1]*cos(u[3]+2*pi/3)-u[2]*sin(u[3]+2*pi/3)
  ABC : Outport  InitialOutput=0
  wires:
  theta/1 -> Mux/2
  Mux1/1 -> ABC/1
  vc/1 -> Mux1/3
  vb/1 -> Mux1/2
  va/1 -> Mux1/1
  DQ/1 -> Mux/1
  Mux/1 -> va/1, vb/1, vc/1

== system wt_blockset_beta/Electrical Machinery/Simulink Blocks  based Models/Squirrel Cage Induction Machine constant parameters/phase ->line ==
  In : Inport
  Mux1 : Mux  Inputs=3
  iab : Fcn  Expr=u(1)-u(2)
  ibc : Fcn  Expr=u(2)-u(3)
  ica : Fcn  Expr=u(3)-u(1)
  Out : Outport
  wires:
  iab/1 -> Mux1/1
  ibc/1 -> Mux1/2
  ica/1 -> Mux1/3
  Mux1/1 -> Out/1
  In/1 -> iab/1, ibc/1, ica/1

== system wt_blockset_beta/Electrical Machinery/Simulink Blocks  based Models/Squirrel Cage  Induction Machine  with Deep Bar Effect/Derivatives ==
  note: DQ Model Of Squirrel-Cage Induction Machine with deep bar effect
  vdqs : Inport
  omega : Inport  Port=2
  Mux : Mux  Inputs=[1 1 1 1 2 1 1 1]
  Selector : Selector  Elements=[7]  InputPortWidth=9
  Selector1 : Selector  Elements=[1 2]  InputPortWidth=9
  didr/dt : Fcn  Expr=((Rs*Lm*u(1))/(Lss*(u(9)+Lm))-Lm*u(7)*u(2)/(u(9)+Lm)-u(8)*u(3)/(u(9)+Lm)-(Lm^2*u(7)*u(4))/(Lss*(u(9)+Lm))-(Lm*u(5))/(Lss*(u(9)+Lm)))/(1-Lm^2/(Lss*(u(9)+Lm)))
  dids/dt : Fcn  Expr=(-Rs*u(1)/Lss+u(7)*u(2)+(Lm*u(8)*u(3))/(Lss*(u(9)+Lm))+Lm*u(7)*u(4)/Lss+u(5)/Lss)/(1-Lm^2/(Lss*(u(9)+Lm)))
  diqr/dt : Fcn  Expr=(Lm*u(7)*u(1)/(u(9)+Lm)+(Rs*Lm*u(2))/(Lss*(u(9)+Lm))+(Lm^2*u(7)*u(3))/(Lss*(u(9)+Lm))-u(8)*u(4)/(u(9)+Lm)-(Lm*u(6))/(Lss*(u(9)+Lm)))/(1-Lm^2/(Lss*(u(9)+Lm)))
  diqs/dt : Fcn  Expr=(-u(7)*u(1)-Rs*u(2)/Lss-Lm*u(7)*u(3)/Lss+(u(8)*Lm*u(4))/(Lss*(u(9)+Lm))+u(6)/Lss)/(1-Lm^2/(Lss*(u(9)+Lm)))
  electromagnetic torque : Fcn  Expr=1.5*Lm*p*(u(2)*u(3)-u(1)*u(4))
  int_1 : Integrator  InitialCondition=x0(1)
  int_2 : Integrator  InitialCondition=x0(2)
  int_3 : Integrator  InitialCondition=x0(3)
  int_4 : Integrator  InitialCondition=x0(4)
  int_5 : Integrator  InitialCondition=x0(5)
  rotor reactance : Fcn  Expr=Lsgmr*(abs(u(1))<=sbd)+(Lsgmr*((kx-1)*abs(u(1))+(1-kx*sbd))/(1-sbd))*(abs(u(1))>sbd)
  rotor resistance : Fcn  Expr=Rr*(abs(u(1))<=sbd)+(Rr*((kr-1)*abs(u(1))+(1-kr*sbd))/(1-sbd))*(abs(u(1))>sbd)
  slip : Fcn  Expr=1-u(1)/omg_base
  idqs : Outport
  Te : Outport  Port=2
  tag scope: theta=global
  wires:
  rotor reactance/1 -> Mux/8
  slip/1 -> rotor reactance/1, rotor resistance/1  "omega_rot"
  rotor resistance/1 -> Mux/7
  Selector1/1 -> idqs/1
  diqs/dt/1 -> int_2/1
  Selector/1 -> int_5/1
  int_5/1 -> [theta]  "theta"
  electromagnetic torque/1 -> Te/1
  diqr/dt/1 -> int_4/1
  didr/dt/1 -> int_3/1
  dids/dt/1 -> int_1/1
  Mux/1 -> Selector1/1, Selector/1, electromagnetic torque/1, diqr/dt/1, didr/dt/1, diqs/dt/1, dids/dt/1
  omega/1 -> Mux/6, slip/1  "omega_rot"
  vdqs/1 -> Mux/5  "vdqs"
  int_4/1 -> Mux/4  "iqr"
  int_3/1 -> Mux/3  "idr"
  int_2/1 -> Mux/2  "iqs"
  int_1/1 -> Mux/1  "ids"

== system wt_blockset_beta/Electrical Machinery/Simulink Blocks  based Models/Squirrel Cage  Induction Machine  with Deep Bar Effect/Subsystem1 ==
  DQ : Inport
  theta : Inport  Port=2
  Mux : Mux  Inputs=[2 1]
  Mux1 : Mux  Inputs=3
  va : Fcn  Expr=u[1]*cos(u[3])-u[2]*sin(u[3])
  vb : Fcn  Expr=u[1]*cos(u[3]-2*pi/3)-u[2]*sin(u[3]-2*pi/3)
  vc : Fcn  Expr=u[1]*cos(u[3]+2*pi/3)-u[2]*sin(u[3]+2*pi/3)
  ABC : Outport  InitialOutput=0
  wires:
  theta/1 -> Mux/2
  Mux1/1 -> ABC/1
  vc/1 -> Mux1/3
  vb/1 -> Mux1/2
  va/1 -> Mux1/1
  DQ/1 -> Mux/1
  Mux/1 -> va/1, vb/1, vc/1

== system wt_blockset_beta/Electrical Machinery/Simulink Blocks  based Models/Squirrel Cage  Induction Machine  with Deep Bar Effect/abc-dq ==
  ABC : Inport
  theta : Inport  Port=2
  Mux : Mux  Inputs=[3 1]
  Mux1 : Mux  Inputs=2
  d : Fcn  Expr=2*(u[1]*cos(u[4])+u[2]*cos(u[4]-2*pi/3)+u[3]*cos(u[4]+2*pi/3))/3
  q : Fcn  Expr=-2*(u[1]*sin(u[4])+u[2]*sin(u[4]-2*pi/3)+u[3]*sin(u[4]+2*pi/3))/3
  DQ : Outport  InitialOutput=0
  wires:
  q/1 -> Mux1/2  "vqs"
  theta/1 -> Mux/2
  Mux1/1 -> DQ/1
  d/1 -> Mux1/1  "vds"
  ABC/1 -> Mux/1
  Mux/1 -> q/1, d/1

== system wt_blockset_beta/Electrical Machinery/Simulink Blocks  based Models/Squirrel Cage  Induction Machine  with Deep Bar Effect/phase ->line ==
  In : Inport
  Mux1 : Mux  Inputs=3
  iab : Fcn  Expr=u(1)-u(2)
  ibc : Fcn  Expr=u(2)-u(3)
  ica : Fcn  Expr=u(3)-u(1)
  Out : Outport
  wires:
  In/1 -> ica/1, ibc/1, iab/1
  Mux1/1 -> Out/1
  ica/1 -> Mux1/3
  ibc/1 -> Mux1/2
  iab/1 -> Mux1/1

== system wt_blockset_beta/Electrical Machinery/Simulink Blocks  based Models/Wound Rotor Induction Machine constant parameters/Subsystem1 ==
  DQ : Inport
  theta : Inport  Port=2
  Mux : Mux  Inputs=[2 1]
  Mux1 : Mux  Inputs=3
  va : Fcn  Expr=u[1]*cos(u[3])-u[2]*sin(u[3])
  vb : Fcn  Expr=u[1]*cos(u[3]-2*pi/3)-u[2]*sin(u[3]-2*pi/3)
  vc : Fcn  Expr=u[1]*cos(u[3]+2*pi/3)-u[2]*sin(u[3]+2*pi/3)
  ABC : Outport  InitialOutput=0
  wires:
  theta/1 -> Mux/2
  Mux1/1 -> ABC/1
  vc/1 -> Mux1/3
  vb/1 -> Mux1/2
  va/1 -> Mux1/1
  DQ/1 -> Mux/1
  Mux/1 -> va/1, vb/1, vc/1

== system wt_blockset_beta/Electrical Machinery/Simulink Blocks  based Models/Wound Rotor Induction Machine constant parameters/Subsystem2 ==
  DQ : Inport
  theta : Inport  Port=2
  Mux : Mux  Inputs=[2 1]
  Mux1 : Mux  Inputs=3
  va : Fcn  Expr=u[1]*cos(u[3])-u[2]*sin(u[3])
  vb : Fcn  Expr=u[1]*cos(u[3]-2*pi/3)-u[2]*sin(u[3]-2*pi/3)
  vc : Fcn  Expr=u[1]*cos(u[3]+2*pi/3)-u[2]*sin(u[3]+2*pi/3)
  ABC : Outport  InitialOutput=0
  wires:
  theta/1 -> Mux/2
  Mux/1 -> vc/1, vb/1, va/1
  DQ/1 -> Mux/1
  va/1 -> Mux1/1
  vb/1 -> Mux1/2
  vc/1 -> Mux1/3
  Mux1/1 -> ABC/1

== system wt_blockset_beta/Electrical Machinery/Simulink Blocks  based Models/Wound Rotor Induction Machine constant parameters/Voltage equations ==
  vdqs : Inport
  vdqr : Inport  Port=2
  omega : Inport  Port=3
  Mux : Mux  Inputs=[1 1 1 1 2 2 1]
  Selector : Selector  Elements=[1 2]  InputPortWidth=9
  Selector1 : Selector  Elements=[3 4]  InputPortWidth=9
  Selector2 : Selector  Elements=[9]  InputPortWidth=9
  didr/dt : Fcn  Expr=(Rs*Lm*u(1)/(Lss*Lsr)-Lm*u(9)*u(2)/Lsr-Rr*u(3)/Lsr-((Lm^2)*u(9)*u(4))/(Lss*Lsr)-Lm*u(5)/(Lss*Lsr)+u(7)/Lsr)/sigma
  dids/dt : Fcn  Expr=(-Rs*u(1)/Lss+u(9)*u(2)+(Lm*Rr*u(3))/(Lss*Lsr)+Lm*u(9)*u(4)/Lss+u(5)/Lss-Lm*u(7)/(Lss*Lsr))/sigma
  diqr/dt : Fcn  Expr=(Lm*u(9)*u(1)/Lsr+Rs*Lm*u(2)/(Lss*Lsr)+((Lm^2)*u(9)*u(3))/(Lss*Lsr)-Rr*u(4)/Lsr-Lm*u(6)/(Lss*Lsr)+u(8)/Lsr)/sigma
  diqs/dt : Fcn  Expr=(-u(9)*u(1)-Rs*u(2)/Lss-Lm*u(9)*u(3)/Lss+(Rr*Lm*u(4))/(Lss*Lsr)+u(6)/Lss-Lm*u(8)/(Lss*Lsr))/sigma
  electromagnetique torque : Fcn  Expr=1.5*Lm*p*(u(2)*u(3)-u(1)*u(4))
  int_1 : Integrator  InitialCondition=x0(1)
  int_2 : Integrator  InitialCondition=x0(2)
  int_3 : Integrator  InitialCondition=x0(3)
  int_4 : Integrator  InitialCondition=x0(4)
  int_5 : Integrator  InitialCondition=x0(5)
  idqs : Outport
  idqr : Outport  Port=2
  Te : Outport  Port=3
  tag scope: theta=global
  wires:
  Selector1/1 -> idqr/1
  Selector/1 -> idqs/1
  vdqr/1 -> Mux/6
  omega/1 -> Mux/7  "omega_rot"
  Selector2/1 -> int_5/1
  int_5/1 -> [theta]  "theta"
  electromagnetique torque/1 -> Te/1
  diqr/dt/1 -> int_4/1  "diqr"
  didr/dt/1 -> int_3/1  "didr"
  diqs/dt/1 -> int_2/1  "diqs"
  dids/dt/1 -> int_1/1  "dids"
  Mux/1 -> Selector1/1, Selector/1, Selector2/1, electromagnetique torque/1, diqr/dt/1, didr/dt/1, diqs/dt/1, dids/dt/1
  vdqs/1 -> Mux/5
  int_4/1 -> Mux/4  "iqr"
  int_3/1 -> Mux/3  "idr"
  int_2/1 -> Mux/2  "iqs"
  int_1/1 -> Mux/1  "ids"

== system wt_blockset_beta/Electrical Machinery/Simulink Blocks  based Models/Wound Rotor Induction Machine constant parameters/abc-dq ==
  ABC : Inport
  theta : Inport  Port=2
  Mux : Mux  Inputs=[3 1]
  Mux1 : Mux  Inputs=2
  d : Fcn  Expr=2*(u[1]*cos(u[4])+u[2]*cos(u[4]-2*pi/3)+u[3]*cos(u[4]+2*pi/3))/3
  q : Fcn  Expr=-2*(u[1]*sin(u[4])+u[2]*sin(u[4]-2*pi/3)+u[3]*sin(u[4]+2*pi/3))/3
  DQ : Outport  InitialOutput=0
  wires:
  q/1 -> Mux1/2  "vqs"
  theta/1 -> Mux/2
  Mux1/1 -> DQ/1
  d/1 -> Mux1/1  "vds"
  ABC/1 -> Mux/1
  Mux/1 -> q/1, d/1

== system wt_blockset_beta/Electrical Machinery/Simulink Blocks  based Models/Wound Rotor Induction Machine constant parameters/abc-dq1 ==
  ABC : Inport
  theta : Inport  Port=2
  Mux : Mux  Inputs=[3 1]
  Mux1 : Mux  Inputs=2
  d : Fcn  Expr=2*(u[1]*cos(u[4])+u[2]*cos(u[4]-2*pi/3)+u[3]*cos(u[4]+2*pi/3))/3
  q : Fcn  Expr=-2*(u[1]*sin(u[4])+u[2]*sin(u[4]-2*pi/3)+u[3]*sin(u[4]+2*pi/3))/3
  DQ : Outport  InitialOutput=0
  wires:
  theta/1 -> Mux/2
  Mux/1 -> d/1, q/1
  ABC/1 -> Mux/1
  d/1 -> Mux1/1  "vdr"
  q/1 -> Mux1/2  "vqr"
  Mux1/1 -> DQ/1

== system wt_blockset_beta/Electrical Machinery/Simulink Blocks  based Models/Wound Rotor Induction Machine with Deep Bar Effect /Subsystem1 ==
  DQ : Inport
  theta : Inport  Port=2
  Mux : Mux  Inputs=[2 1]
  Mux1 : Mux  Inputs=3
  va : Fcn  Expr=u[1]*cos(u[3])-u[2]*sin(u[3])
  vb : Fcn  Expr=u[1]*cos(u[3]-2*pi/3)-u[2]*sin(u[3]-2*pi/3)
  vc : Fcn  Expr=u[1]*cos(u[3]+2*pi/3)-u[2]*sin(u[3]+2*pi/3)
  ABC : Outport  InitialOutput=0
  wires:
  Mux/1 -> vc/1, vb/1, va/1
  DQ/1 -> Mux/1
  va/1 -> Mux1/1
  vb/1 -> Mux1/2
  vc/1 -> Mux1/3
  Mux1/1 -> ABC/1
  theta/1 -> Mux/2

== system wt_blockset_beta/Electrical Machinery/Simulink Blocks  based Models/Wound Rotor Induction Machine with Deep Bar Effect /Subsystem2 ==
  DQ : Inport
  theta : Inport  Port=2
  Mux : Mux  Inputs=[2 1]
  Mux1 : Mux  Inputs=3
  va : Fcn  Expr=u[1]*cos(u[3])-u[2]*sin(u[3])
  vb : Fcn  Expr=u[1]*cos(u[3]-2*pi/3)-u[2]*sin(u[3]-2*pi/3)
  vc : Fcn  Expr=u[1]*cos(u[3]+2*pi/3)-u[2]*sin(u[3]+2*pi/3)
  ABC : Outport  InitialOutput=0
  wires:
  Mux1/1 -> ABC/1
  vc/1 -> Mux1/3
  vb/1 -> Mux1/2
  va/1 -> Mux1/1
  DQ/1 -> Mux/1
  Mux/1 -> va/1, vb/1, vc/1
  theta/1 -> Mux/2

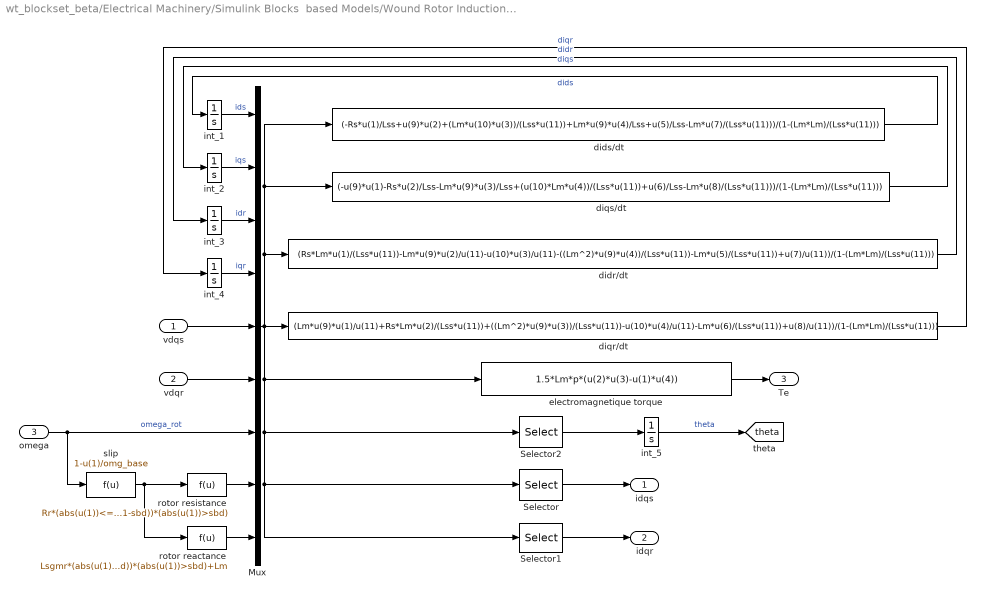
== system wt_blockset_beta/Electrical Machinery/Simulink Blocks  based Models/Wound Rotor Induction Machine with Deep Bar Effect /Voltage equations ==
  vdqs : Inport
  vdqr : Inport  Port=2
  omega : Inport  Port=3
  Mux : Mux  Inputs=[1 1 1 1 2 2 1 1 1]
  Selector : Selector  Elements=[1 2]  InputPortWidth=11
  Selector1 : Selector  Elements=[3 4]  InputPortWidth=11
  Selector2 : Selector  Elements=[9]  InputPortWidth=11
  didr/dt : Fcn  Expr=(Rs*Lm*u(1)/(Lss*u(11))-Lm*u(9)*u(2)/u(11)-u(10)*u(3)/u(11)-((Lm^2)*u(9)*u(4))/(Lss*u(11))-Lm*u(5)/(Lss*u(11))+u(7)/u(11))/(1-(Lm*Lm)/(Lss*u(11)))
  dids/dt : Fcn  Expr=(-Rs*u(1)/Lss+u(9)*u(2)+(Lm*u(10)*u(3))/(Lss*u(11))+Lm*u(9)*u(4)/Lss+u(5)/Lss-Lm*u(7)/(Lss*u(11)))/(1-(Lm*Lm)/(Lss*u(11)))
  diqr/dt : Fcn  Expr=(Lm*u(9)*u(1)/u(11)+Rs*Lm*u(2)/(Lss*u(11))+((Lm^2)*u(9)*u(3))/(Lss*u(11))-u(10)*u(4)/u(11)-Lm*u(6)/(Lss*u(11))+u(8)/u(11))/(1-(Lm*Lm)/(Lss*u(11)))
  diqs/dt : Fcn  Expr=(-u(9)*u(1)-Rs*u(2)/Lss-Lm*u(9)*u(3)/Lss+(u(10)*Lm*u(4))/(Lss*u(11))+u(6)/Lss-Lm*u(8)/(Lss*u(11)))/(1-(Lm*Lm)/(Lss*u(11)))
  electromagnetique torque : Fcn  Expr=1.5*Lm*p*(u(2)*u(3)-u(1)*u(4))
  int_1 : Integrator  InitialCondition=x0(1)
  int_2 : Integrator  InitialCondition=x0(2)
  int_3 : Integrator  InitialCondition=x0(3)
  int_4 : Integrator  InitialCondition=x0(4)
  int_5 : Integrator  InitialCondition=x0(5)
  rotor reactance : Fcn  Expr=Lsgmr*(abs(u(1))<=sbd)+(Lsgmr*((kx-1)*abs(u(1))+(1-kx*sbd))/(1-sbd))*(abs(u(1))>sbd)+Lm
  rotor resistance : Fcn  Expr=Rr*(abs(u(1))<=sbd)+(Rr*((kr-1)*abs(u(1))+(1-kr*sbd))/(1-sbd))*(abs(u(1))>sbd)
  slip : Fcn  Expr=1-u(1)/omg_base
  idqs : Outport
  idqr : Outport  Port=2
  Te : Outport  Port=3
  tag scope: theta=global
  wires:
  int_1/1 -> Mux/1  "ids"
  int_2/1 -> Mux/2  "iqs"
  int_3/1 -> Mux/3  "idr"
  int_4/1 -> Mux/4  "iqr"
  vdqs/1 -> Mux/5
  dids/dt/1 -> int_1/1  "dids"
  diqs/dt/1 -> int_2/1  "diqs"
  didr/dt/1 -> int_3/1  "didr"
  diqr/dt/1 -> int_4/1  "diqr"
  electromagnetique torque/1 -> Te/1
  int_5/1 -> [theta]  "theta"
  Selector2/1 -> int_5/1
  omega/1 -> Mux/7, slip/1  "omega_rot"
  vdqr/1 -> Mux/6
  Selector/1 -> idqs/1
  Selector1/1 -> idqr/1
  slip/1 -> rotor resistance/1, rotor reactance/1
  rotor resistance/1 -> Mux/8
  rotor reactance/1 -> Mux/9
  Mux/1 -> diqr/dt/1, didr/dt/1, diqs/dt/1, dids/dt/1, electromagnetique torque/1, Selector2/1, Selector/1, Selector1/1

== system wt_blockset_beta/Electrical Machinery/Simulink Blocks  based Models/Wound Rotor Induction Machine with Deep Bar Effect /abc-dq ==
  ABC : Inport
  theta : Inport  Port=2
  Mux : Mux  Inputs=[3 1]
  Mux1 : Mux  Inputs=2
  d : Fcn  Expr=2*(u[1]*cos(u[4])+u[2]*cos(u[4]-2*pi/3)+u[3]*cos(u[4]+2*pi/3))/3
  q : Fcn  Expr=-2*(u[1]*sin(u[4])+u[2]*sin(u[4]-2*pi/3)+u[3]*sin(u[4]+2*pi/3))/3
  DQ : Outport  InitialOutput=0
  wires:
  Mux/1 -> d/1, q/1
  ABC/1 -> Mux/1
  d/1 -> Mux1/1  "vds"
  Mux1/1 -> DQ/1
  theta/1 -> Mux/2
  q/1 -> Mux1/2  "vqs"

== system wt_blockset_beta/Electrical Machinery/Simulink Blocks  based Models/Wound Rotor Induction Machine with Deep Bar Effect /abc-dq1 ==
  ABC : Inport
  theta : Inport  Port=2
  Mux : Mux  Inputs=[3 1]
  Mux1 : Mux  Inputs=2
  d : Fcn  Expr=2*(u[1]*cos(u[4])+u[2]*cos(u[4]-2*pi/3)+u[3]*cos(u[4]+2*pi/3))/3
  q : Fcn  Expr=-2*(u[1]*sin(u[4])+u[2]*sin(u[4]-2*pi/3)+u[3]*sin(u[4]+2*pi/3))/3
  DQ : Outport  InitialOutput=0
  wires:
  Mux1/1 -> DQ/1
  q/1 -> Mux1/2  "vqr"
  d/1 -> Mux1/1  "vdr"
  ABC/1 -> Mux/1
  Mux/1 -> q/1, d/1
  theta/1 -> Mux/2

== system wt_blockset_beta/Measurements/power spectra/Spectrum Scope/Optional Buffering ==
  In : Inport
  Buffer : Mux  Inputs=1
  Out : Outport  InitialOutput=0
  wires:
  Buffer/1 -> Out/1
  In/1 -> Buffer/1

== system wt_blockset_beta/Mechanical Components/Wind Model SB-2/3rd_Harmonic_Filter1/3rd harmonic Filter ==
  avg_wind : Inport
  In : Inport  Port=2
  Coefficients : Subsystem
  Integrator : Integrator  Orientation=up
  Integrator1 : Integrator  Orientation=up
  Product : Product  SaturateOnIntegerOverflow=on
  Product1 : Product  SaturateOnIntegerOverflow=on
  Product2 : Product  Orientation=left  SaturateOnIntegerOverflow=on
  Product3 : Product  Orientation=left  SaturateOnIntegerOverflow=on
  Sum1 : Sum  Orientation=up  Inputs=++-  SaturateOnIntegerOverflow=on
  Sum2 : Sum  Orientation=up  Inputs=+|-  SaturateOnIntegerOverflow=on
  Out : Outport
  wires:
  Integrator/1 -> Product2/1, Product3/1, Out/1
  Sum1/1 -> Integrator/1
  Product/1 -> Sum1/1
  Integrator1/1 -> Sum1/2
  Product2/1 -> Sum1/3
  Sum2/1 -> Integrator1/1
  Product3/1 -> Sum2/2
  Product1/1 -> Sum2/1
  In/1 -> Product/1, Product1/1
  [BD] -> Product/2
  [CD] -> Product1/2
  [ED] -> Product2/2
  [FD] -> Product3/2
  Coefficients/1(BD) -> [BD]
  Coefficients/2(CD) -> [CD]
  Coefficients/3(ED) -> [ED]
  Coefficients/4(FD) -> [FD]
  avg_wind/1 -> Coefficients/1(avg_wind)

== system wt_blockset_beta/Mechanical Components/Wind Model SB-2/3rd_Harmonic_Filter2/3rd harmonic Filter ==
  avg_wind : Inport
  In : Inport  Port=2
  Coefficients : Subsystem
  Integrator : Integrator  Orientation=up
  Integrator1 : Integrator  Orientation=up
  Product : Product  SaturateOnIntegerOverflow=on
  Product1 : Product  SaturateOnIntegerOverflow=on
  Product2 : Product  Orientation=left  SaturateOnIntegerOverflow=on
  Product3 : Product  Orientation=left  SaturateOnIntegerOverflow=on
  Sum1 : Sum  Orientation=up  Inputs=++-  SaturateOnIntegerOverflow=on
  Sum2 : Sum  Orientation=up  Inputs=+|-  SaturateOnIntegerOverflow=on
  Out : Outport
  wires:
  avg_wind/1 -> Coefficients/1(avg_wind)
  Coefficients/4(FD) -> [FD]
  Coefficients/3(ED) -> [ED]
  Coefficients/2(CD) -> [CD]
  Coefficients/1(BD) -> [BD]
  [FD] -> Product3/2
  [ED] -> Product2/2
  [CD] -> Product1/2
  [BD] -> Product/2
  In/1 -> Product1/1, Product/1
  Product1/1 -> Sum2/1
  Product3/1 -> Sum2/2
  Sum2/1 -> Integrator1/1
  Product2/1 -> Sum1/3
  Integrator1/1 -> Sum1/2
  Product/1 -> Sum1/1
  Sum1/1 -> Integrator/1
  Integrator/1 -> Out/1, Product3/1, Product2/1

== system wt_blockset_beta/Mechanical Components/Wind Model SB-2/Kaimal_Filter_1/Kaimal Filter ==
  avg_wind : Inport
  In : Inport  Port=2
  A/D : Gain  Gain=0.0182/1.3463  SaturateOnIntegerOverflow=on
  Coefficients : Subsystem
  Integrator : Integrator  Orientation=up
  Integrator1 : Integrator  Orientation=up
  Product : Product  SaturateOnIntegerOverflow=on
  Product1 : Product  SaturateOnIntegerOverflow=on
  Product2 : Product  Orientation=left  SaturateOnIntegerOverflow=on
  Product3 : Product  Orientation=left  SaturateOnIntegerOverflow=on
  Sum : Sum  Inputs=|++  SaturateOnIntegerOverflow=on
  Sum1 : Sum  Orientation=up  Inputs=++-  SaturateOnIntegerOverflow=on
  Sum2 : Sum  Orientation=up  Inputs=+|-  SaturateOnIntegerOverflow=on
  Out : Outport
  wires:
  A/D/1 -> Sum/1
  Integrator/1 -> Sum/2
  Sum1/1 -> Integrator/1
  Product/1 -> Sum1/1
  Integrator1/1 -> Sum1/2
  Product2/1 -> Sum1/3
  Sum2/1 -> Integrator1/1
  Product3/1 -> Sum2/2
  Product1/1 -> Sum2/1
  Sum/1 -> Product2/1, Product3/1, Out/1
  In/1 -> A/D/1, Product/1, Product1/1
  [BD] -> Product/2
  [CD] -> Product1/2
  [ED] -> Product2/2
  [FD] -> Product3/2
  Coefficients/1(BD) -> [BD]
  Coefficients/2(CD) -> [CD]
  Coefficients/3(ED) -> [ED]
  Coefficients/4(FD) -> [FD]
  avg_wind/1 -> Coefficients/1(avg_wind)
